simulink model "project_sim"  (R2025a)
settings: Solver=VariableStepAuto  StartTime=0.0  StopTime=120  FixedStep=.05  RelTol=1e-3  EnableMultiTasking=on
values from neighbouring files (symbols this model uses):
  A = double(subs(A, {m, I, l, beta, g}, {m_use, I_use, l_use, beta_use, g_use}))    [derivation_project.m]
  B = double(subs(B, {m, I, l, beta, g}, {m_use, I_use, l_use, beta_use, g_use}))    [derivation_project.m]
  C = [1 0 0 0 0 0; 0 1 0 0 0 0]    [derivation_project.m]
  G1 = inv(C * inv(B*K - A) * B)    [derivation_project.m]
  G2 = ((C * ((B*K - A)^-2) * B)) / ( (C * ((B*K - A)^-1)*B)^2 )    [derivation_project.m]
  g_use = 9.81    [derivation_project.m]
  K = subs(K,{x,y,theta,xdot,ydot,thetadot, Tl, Tr},{x_op, y_op, theta_op, dx_op, dy_op, dtheta_op, Tl_op, Tr_op})    [derivation_project.m]
  L = transpose(L_t)    [derivation_project.m]
  m_use = 1.4    [derivation_project.m]
libraries: simulink x2
settings Model: Creator=Caleb Rucker  LastModifiedBy=maxho
settings SolverCC: AlgebraicLoopSolver=TrustRegion
settings DataIOCC: LimitDataPoints=on  SaveFormat=Array  ReturnWorkspaceOutputs=off
settings OptimizationCC: LifeSpan=inf
settings DebuggingCC: SolverPrmCheckMsg=warning  UnconnectedInputMsg=warning  UnconnectedOutputMsg=warning  UnconnectedLineMsg=warning  SFUnexpectedBacktrackingDiag=warning  SFNoUnconditionalDefaultTransitionDiag=warning  SFExecutionAtInitializationDiag=none  ArithmeticOperatorsInVariantConditions=warning
settings HardwareCC: ProdBitPerPointer=32.0  ProdBitPerSizeT=32.0  ProdBitPerPtrDiffT=32.0  ProdLargestAtomicFloat=None  ProdIntDivRoundTo=Undefined  ProdEndianess=Unspecified  ProdWordSize=32.0  ProdHWDeviceType=32-bit Generic
settings ModelReferenceCC: EnableRefExpFcnMdlSchedulingChecks=on  PropagateSignalLabelsOutOfModel=off
settings SFSimCC: SimUseLocalCustomCode=off  CustomCodeUndefinedFunction=UseInterfaceOnly
settings RTWCC: RTWUseLocalCustomCode=off  GPUComputeCapability=3.5  DLArmComputeVersion=19.05
settings CodeAppCC: StateflowObjectComments=on
settings GRTTargetCC: TargetLangStandard=C89/C90 (ANSI)
settings ConfigComp: CovMetricSettings=dw  CovSaveCumulativeToWorkspaceVar=on  CovSaveSingleToWorkspaceVar=on  CovExternalEMLEnable=off  CovSFcnEnable=off

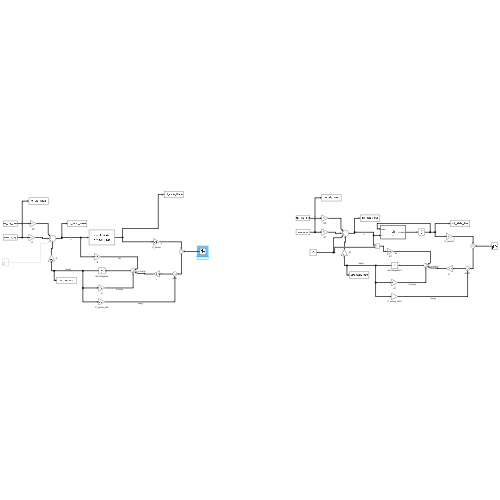
[thumbnail: Simulink's stored preview of the top-level diagram]
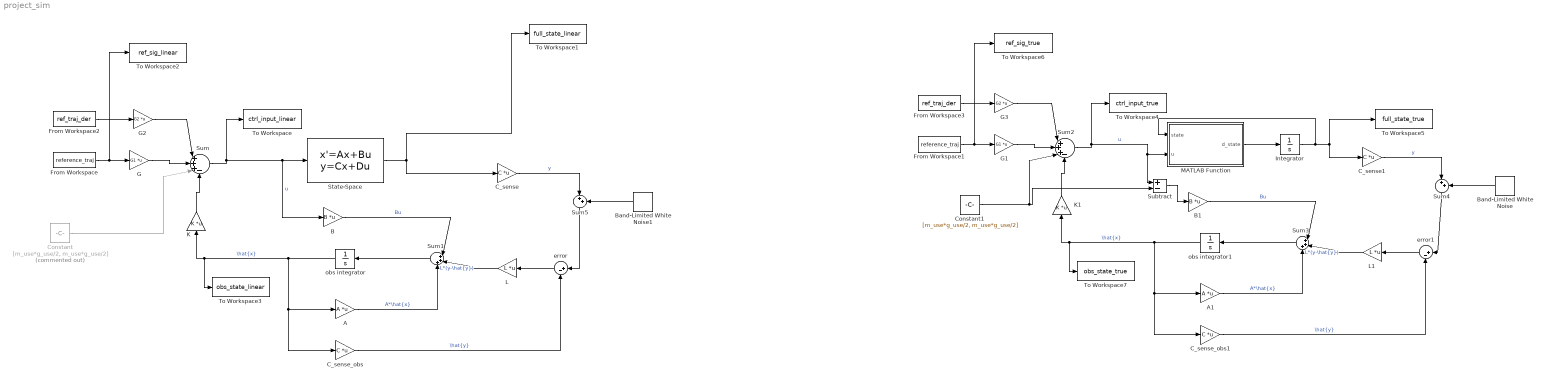
== system project_sim ==
  A : Gain  Gain=A  Multiplication=Matrix(K*u)
  A1 : Gain  Gain=A  Multiplication=Matrix(K*u)
  B : Gain  Gain=B  Multiplication=Matrix(K*u)
  B1 : Gain  Gain=B  Multiplication=Matrix(K*u)
  Band-Limited White Noise : simulink/Sources/Band-Limited White Noise  Cov=sens_power  Ts=0.01  seed=[23341]
  Band-Limited White Noise1 : simulink/Sources/Band-Limited White Noise  Cov=sens_power  Ts=0.01  seed=[23341]
  C_sense : Gain  Gain=C  Multiplication=Matrix(K*u)
  C_sense1 : Gain  Gain=C  Multiplication=Matrix(K*u)
  C_sense_obs : Gain  Gain=C  Multiplication=Matrix(K*u)
  C_sense_obs1 : Gain  Gain=C  Multiplication=Matrix(K*u)
  Constant : Constant  Commented=on  Value=[m_use*g_use/2, m_use*g_use/2]
  Constant1 : Constant  Value=[m_use*g_use/2, m_use*g_use/2]
  From Workspace : FromWorkspace  VariableName=reference_traj  OutDataTypeStr=double  SampleTime=0.01  OutputAfterFinalValue=Setting to zero
  From Workspace1 : FromWorkspace  VariableName=reference_traj  OutDataTypeStr=double  SampleTime=0.01  OutputAfterFinalValue=Setting to zero
  From Workspace2 : FromWorkspace  VariableName=ref_traj_der  OutDataTypeStr=double  SampleTime=0.01
  From Workspace3 : FromWorkspace  VariableName=ref_traj_der  OutDataTypeStr=double  SampleTime=0.01
  G : Gain  Gain=G1  Multiplication=Matrix(K*u)
  G1 : Gain  Gain=G1  Multiplication=Matrix(K*u)
  G2 : Gain  Gain=G2  Multiplication=Matrix(K*u)
  G3 : Gain  Gain=G2  Multiplication=Matrix(K*u)
  Integrator : Integrator  InitialCondition=[1.0; 0.4; 0; 0.0; 0; 0]
  K : Gain  Gain=K  Multiplication=Matrix(K*u)
  K1 : Gain  Gain=K  Multiplication=Matrix(K*u)
  L : Gain  Gain=L  Multiplication=Matrix(K*u)
  L1 : Gain  Gain=L  Multiplication=Matrix(K*u)
  MATLAB Function : MATLAB Function  TreatAsAtomicUnit=on
  State-Space : StateSpace  A=A  B=B  C=eye(6)  D=zeros(6,2)  InitialCondition=[1.0; 0.4; 0; 0.0; 0; 0]
  Subtract : Sum  Inputs=+-
  Sum : Sum  Inputs=|+++-
  Sum1 : Sum  Inputs=|+++
  Sum2 : Sum  Inputs=|+++-
  Sum3 : Sum  Inputs=|+++
  Sum4 : Sum  Inputs=|++
  Sum5 : Sum  Inputs=|++
  To Workspace : ToWorkspace  VariableName=ctrl_input_linear  SaveFormat=Timeseries  SampleTime=-1
  To Workspace1 : ToWorkspace  VariableName=full_state_linear  SaveFormat=Timeseries  SampleTime=-1
  To Workspace2 : ToWorkspace  VariableName=ref_sig_linear  SaveFormat=Timeseries  SampleTime=-1
  To Workspace3 : ToWorkspace  VariableName=obs_state_linear  SaveFormat=Timeseries  SampleTime=-1
  To Workspace4 : ToWorkspace  VariableName=ctrl_input_true  SaveFormat=Timeseries  SampleTime=-1
  To Workspace5 : ToWorkspace  VariableName=full_state_true  SaveFormat=Timeseries  SampleTime=-1
  To Workspace6 : ToWorkspace  VariableName=ref_sig_true  SaveFormat=Timeseries  SampleTime=-1
  To Workspace7 : ToWorkspace  VariableName=obs_state_true  SaveFormat=Timeseries  SampleTime=-1
  error : Sum  Inputs=|+-
  error1 : Sum  Inputs=|+-
  obs integrator : Integrator  InitialCondition=[0.9, 0.3, 0, 0, 0, 0]
  obs integrator1 : Integrator  InitialCondition=[0.9; 0.3; 0; 0; 0; 0]
  wires:
  State-Space/1 -> To Workspace1/1, C_sense/1
  From Workspace/1 -> To Workspace2/1, G/1
  Sum/1 -> To Workspace/1, State-Space/1, B/1  "u"
  obs integrator/1 -> C_sense_obs/1, A/1, K/1, To Workspace3/1  "\\hat{x}"
  A/1 -> Sum1/3  "A*\\hat{x}"
  B/1 -> Sum1/1  "Bu"
  C_sense_obs/1 -> error/2  "\\hat{y}"
  error/1 -> L/1
  L/1 -> Sum1/2  "L*(y-\\hat{y})"
  Sum1/1 -> obs integrator/1
  From Workspace1/1 -> To Workspace6/1, G1/1
  A1/1 -> Sum3/3  "A*\\hat{x}"
  MATLAB Function/1(d_state) -> Integrator/1
  Sum2/1 -> To Workspace4/1, Subtract/1, MATLAB Function/2(u)  "u"
  L1/1 -> Sum3/2  "L*(y-\\hat{y})"
  error1/1 -> L1/1
  obs integrator1/1 -> C_sense_obs1/1, A1/1, K1/1, To Workspace7/1  "\\hat{x}"
  C_sense_obs1/1 -> error1/2  "\\hat{y}"
  Sum3/1 -> obs integrator1/1
  Integrator/1 -> MATLAB Function/1(state), To Workspace5/1, C_sense1/1
  Constant1/1 -> Sum2/3, Subtract/2
  B1/1 -> Sum3/1  "Bu"
  Subtract/1 -> B1/1
  K/1 -> Sum/4
  Constant/1 -> Sum/3
  G/1 -> Sum/2
  From Workspace2/1 -> G2/1
  G2/1 -> Sum/1
  K1/1 -> Sum2/4
  G1/1 -> Sum2/2
  From Workspace3/1 -> G3/1
  G3/1 -> Sum2/1
  C_sense1/1 -> Sum4/1  "y"
  Sum4/1 -> error1/1
  Band-Limited White Noise/1 -> Sum4/2
  Band-Limited White Noise1/1 -> Sum5/2
  C_sense/1 -> Sum5/1  "y"
  Sum5/1 -> error/1

== matlab function project_sim/MATLAB Function ==
  data: state input; u input; d_state output
function d_state = fcn(state, u)

    Tl = u(1);
    Tr = u(2);

    m = 1.4;
    I = 0.0211;
    l = 0.159;
    beta = 0.1365;
    g = 9.81;
    
    theta = state(3);
    xdot = state(4);
    ydot = state(5);
    thetadot = state(6);

    xddot = (-(Tl + Tr)*sin(theta) - beta * xdot * sqrt(xdot^2 + ydot^2)) / m;
    yddot = (((Tl + Tr) * cos(theta) - beta * ydot * sqrt(xdot^2 + ydot^2)) / m) - g;
    thetaddot = (Tr - Tl) * l / I;

    d_state = [xdot; ydot; thetadot; xddot; yddot; thetaddot];
